simulink model "analiseLongitudinal_NL"  (R2016a)
settings: Solver=ode4  StartTime=0.0  StopTime=300  FixedStep=0.01  RelTol=1e-3
undefined symbols (not defined in the file): Ch, Ctheta, CVt, degtorad, Kh, Kq, Ktheta, KVt, Ue, Xe
libraries: simulink x13
settings Model: PauseTimes=50  Creator=Marcelo Henrique  LastModifiedBy=Marcelo
settings DataIOCC: LimitDataPoints=on  SaveFormat=Array
settings DebuggingCC: AlgebraicLoopMsg=none  UnderspecifiedInitializationDetection=Classic  MergeDetectMultiDrivingBlocksExec=none  StateNameClashWarn=warning
settings HardwareCC: ProdBitPerPointer=32  ProdLargestAtomicFloat=None  ProdIntDivRoundTo=Undefined  ProdEndianess=Unspecified  ProdWordSize=32  ProdHWDeviceType=32-bit Generic
settings ModelReferenceCC: PropagateSignalLabelsOutOfModel=off
settings RTWCC: CustomInclude=C:\Users\Marcelo\Desktop\cobem17\ctrl\matlab\mdl
settings ConfigComp: CovModelRefEnable=Off

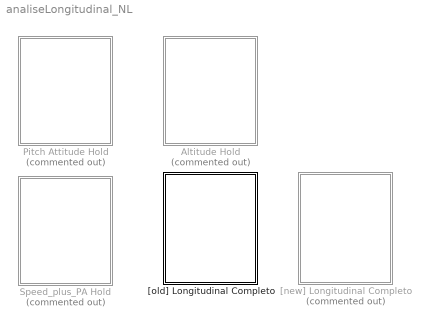
== system analiseLongitudinal_NL ==
  Altitude Hold : Subsystem  Commented=on
  Pitch Attitude Hold : Subsystem  Commented=on
  Speed_plus_PA Hold : Subsystem  Commented=on
  "[new] Longitudinal Completo" : Subsystem  Commented=on
  "[old] Longitudinal Completo" : Subsystem

== system analiseLongitudinal_NL/Altitude Hold ==
  Step1 : Step  Time=20  Before=-Xe(12)  After=-Xe(12)+5  SampleTime=0
  "[Aeronave]" : Subsystem
  "[Controle]" : Subsystem
  "[Navegação]" : Subsystem
  wires:
  "[Aeronave]"/1(Y) -> "[Navegação]"/1(Y)
  "[Navegação]"/1(Yn) -> "[Controle]"/2(Yn)
  Step1/1 -> "[Controle]"/1(Ref)
  "[Controle]"/1(du) -> "[Aeronave]"/1(du)

== system analiseLongitudinal_NL/Pitch Attitude Hold ==
  Step1 : Step  Time=20  Before=Xe(8)  After=degtorad(5)+(Xe(8))  SampleTime=0
  "[Aeronave]" : Subsystem
  "[Controle]" : Subsystem
  "[Navegação]" : Subsystem
  wires:
  "[Aeronave]"/1(Y) -> "[Navegação]"/1(Y)
  "[Controle]"/1(du) -> "[Aeronave]"/1(du)
  "[Navegação]"/1(Yn) -> "[Controle]"/2(Yn)
  Step1/1 -> "[Controle]"/1(Ref)

== system analiseLongitudinal_NL/Speed_plus_PA Hold ==
  Mux : Mux  Inputs=2
  VT_r : Step  Time=0  Before=norm(Xe(1:3))  After=norm(Xe(1:3))  SampleTime=0
  "[Aeronave]" : Subsystem
  "[Controle]" : Subsystem
  "[Navegação]" : Subsystem
  theta_r : Step  Time=20  Before=Xe(8)  After=degtorad(5)+(Xe(8))  SampleTime=0
  wires:
  "[Aeronave]"/1(Y) -> "[Navegação]"/1(Y)
  "[Controle]"/1(du) -> "[Aeronave]"/1(du)
  "[Navegação]"/1(Yn) -> "[Controle]"/2(Yn)
  VT_r/1 -> Mux/1
  theta_r/1 -> Mux/2
  Mux/1 -> "[Controle]"/1(Ref)

== system analiseLongitudinal_NL/[new] Longitudinal Completo ==
  Add : Sum  Inputs=+++
  Mux : Mux  Inputs=2
  Step : Step  Time=50  Before=-Xe(12)  After=-Xe(12)+40  SampleTime=0
  Step1 : Step  Time=150  After=-80  SampleTime=0
  Step2 : Step  Time=250  After=40  SampleTime=0
  Unit Delay : UnitDelay  SampleTime=-1
  VT_r : Step  Time=0  Before=norm(Xe(1:3))  After=norm(Xe(1:3))  SampleTime=0
  "[Aeronave]" : Subsystem
  "[Controle]" : Subsystem
  "[Navegação]" : Subsystem
  wires:
  VT_r/1 -> Mux/1
  Mux/1 -> "[Controle]"/1(U)
  "[Aeronave]"/1(Y) -> "[Navegação]"/1(Y)
  "[Controle]"/1(du) -> Unit Delay/1
  "[Navegação]"/1(Yn) -> "[Controle]"/2(Y)
  Add/1 -> Mux/2  "h_r"
  Step/1 -> Add/1
  Step1/1 -> Add/2
  Step2/1 -> Add/3
  Unit Delay/1 -> "[Aeronave]"/1(du)

== system analiseLongitudinal_NL/[old] Longitudinal Completo ==
  Add : Sum  Inputs=+++
  Mux : Mux  Inputs=2
  Step : Step  Time=50  Before=-Xe(12)  After=-Xe(12)+25  SampleTime=0
  Step1 : Step  Time=150  After=-50  SampleTime=0
  Step2 : Step  Time=250  After=25  SampleTime=0
  VT_r : Step  Time=0  Before=norm(Xe(1:3))  After=norm(Xe(1:3))  SampleTime=0
  "[Aeronave]" : Subsystem
  "[Controle]" : Subsystem
  "[Navegação]" : Subsystem
  wires:
  VT_r/1 -> Mux/1
  Mux/1 -> "[Controle]"/1(U)
  "[Aeronave]"/1(Y) -> "[Navegação]"/1(Y)
  "[Navegação]"/1(Yn) -> "[Controle]"/2(Y)
  Add/1 -> Mux/2  "h_r"
  Step/1 -> Add/1
  Step1/1 -> Add/2
  Step2/1 -> Add/3
  "[Controle]"/1(du) -> "[Aeronave]"/1(du)

== system analiseLongitudinal_NL/Altitude Hold/[Aeronave] ==
  du : Inport
  Entradas equilibrio : Constant  Value=Ue
  S-Function : S-Function  FunctionName=sfunction_piper  Parameters=par_gen,par_aero,par_prop, Xe  SFunctionDeploymentMode=off  EnableBusSupport=off
  Sum1 : Sum
  To Workspace1 : ToWorkspace  VariableName=NLU  SaveFormat=Timeseries  SampleTime=-1
  Y : Outport
  wires:
  S-Function/1 -> Y/1
  Entradas equilibrio/1 -> Sum1/2
  du/1 -> Sum1/1
  Sum1/1 -> To Workspace1/1, S-Function/1

== system analiseLongitudinal_NL/Altitude Hold/[Controle] ==
  Ref : Inport
  Yn : Inport  Port=2
  Controlador Elevator : Subsystem
  Gain8 : Gain  Gain=180/pi
  Mux : Mux
  To Workspace1 : ToWorkspace  VariableName=NLstep  SaveFormat=Timeseries  SampleTime=-1
  d_aileron : Constant  Value=0
  d_rudder : Constant  Value=0
  d_throttle : Constant  Value=0
  delta_e : Scope
  du : Outport
  wires:
  Yn/1 -> Controlador Elevator/2(Yn)
  Mux/1 -> du/1
  d_aileron/1 -> Mux/3
  d_rudder/1 -> Mux/4
  Gain8/1 -> delta_e/1
  Controlador Elevator/1(d_elevator) -> Gain8/1, Mux/2
  d_throttle/1 -> Mux/1
  Ref/1 -> To Workspace1/1, Controlador Elevator/1(h_r)

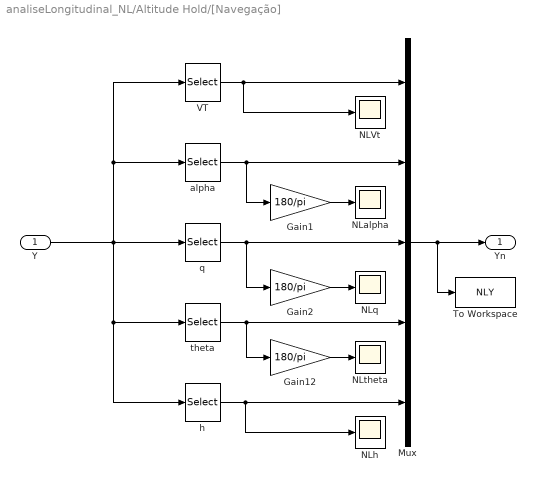
== system analiseLongitudinal_NL/Altitude Hold/[Navegação] ==
  Y : Inport
  Gain1 : Gain  Gain=180/pi
  Gain12 : Gain  Gain=180/pi
  Gain2 : Gain  Gain=180/pi
  Mux : Mux  Inputs=5
  NLVt : Scope
  NLalpha : Scope
  NLh : Scope
  NLq : Scope
  NLtheta : Scope
  To Workspace : ToWorkspace  VariableName=NLY  SaveFormat=Timeseries  SampleTime=-1
  VT : Selector  InputPortWidth=12  IndexOptions=Index vector (dialog)  Indices=[1]  OutputSizes=1
  alpha : Selector  InputPortWidth=12  IndexOptions=Index vector (dialog)  Indices=[2]  OutputSizes=1
  h : Selector  InputPortWidth=12  IndexOptions=Index vector (dialog)  Indices=[12]  OutputSizes=1
  q : Selector  InputPortWidth=12  IndexOptions=Index vector (dialog)  Indices=[5]  OutputSizes=1
  theta : Selector  InputPortWidth=12  IndexOptions=Index vector (dialog)  Indices=[8]  OutputSizes=1
  Yn : Outport
  wires:
  Y/1 -> h/1, theta/1, VT/1, alpha/1, q/1
  Gain12/1 -> NLtheta/1
  VT/1 -> NLVt/1, Mux/1
  theta/1 -> Gain12/1, Mux/4
  h/1 -> NLh/1, Mux/5
  Gain1/1 -> NLalpha/1
  alpha/1 -> Gain1/1, Mux/2
  Gain2/1 -> NLq/1
  q/1 -> Gain2/1, Mux/3
  Mux/1 -> To Workspace/1, Yn/1

== system analiseLongitudinal_NL/Pitch Attitude Hold/[Aeronave] ==
  du : Inport
  Entradas equilibrio : Constant  Value=Ue
  S-Function : S-Function  FunctionName=sfunction_piper  Parameters=par_gen,par_aero,par_prop, Xe  SFunctionDeploymentMode=off  EnableBusSupport=off
  Sum3 : Sum
  To Workspace1 : ToWorkspace  VariableName=NLU  SaveFormat=Timeseries  SampleTime=-1
  Y : Outport
  wires:
  Sum3/1 -> S-Function/1, To Workspace1/1
  du/1 -> Sum3/1
  S-Function/1 -> Y/1
  Entradas equilibrio/1 -> Sum3/2

== system analiseLongitudinal_NL/Pitch Attitude Hold/[Controle] ==
  Ref : Inport
  Yn : Inport  Port=2
  Controlador Elevator : Subsystem
  Gain8 : Gain  Gain=180/pi
  Mux : Mux
  To Workspace1 : ToWorkspace  VariableName=NLstep  SaveFormat=Timeseries  SampleTime=-1
  d_aileron : Constant  Value=0
  d_rudder : Constant  Value=0
  d_throttle : Constant  Value=0
  delta_e : Scope
  du : Outport
  wires:
  Yn/1 -> Controlador Elevator/2(Yn)
  Mux/1 -> du/1
  d_aileron/1 -> Mux/3
  d_rudder/1 -> Mux/4
  Gain8/1 -> delta_e/1
  Controlador Elevator/1(d_elevator) -> Gain8/1, Mux/2
  d_throttle/1 -> Mux/1
  Ref/1 -> To Workspace1/1, Controlador Elevator/1(theta_r)

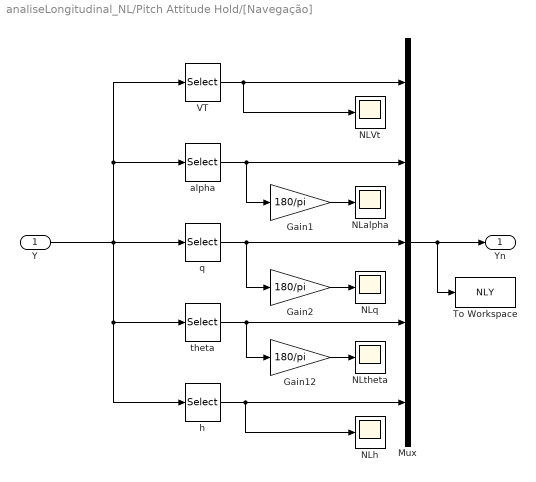
== system analiseLongitudinal_NL/Pitch Attitude Hold/[Navegação] ==
  Y : Inport
  Gain1 : Gain  Gain=180/pi
  Gain12 : Gain  Gain=180/pi
  Gain2 : Gain  Gain=180/pi
  Mux : Mux  Inputs=5
  NLVt : Scope
  NLalpha : Scope
  NLh : Scope
  NLq : Scope
  NLtheta : Scope
  To Workspace : ToWorkspace  VariableName=NLY  SaveFormat=Timeseries  SampleTime=-1
  VT : Selector  InputPortWidth=12  IndexOptions=Index vector (dialog)  Indices=[1]  OutputSizes=1
  alpha : Selector  InputPortWidth=12  IndexOptions=Index vector (dialog)  Indices=[2]  OutputSizes=1
  h : Selector  InputPortWidth=12  IndexOptions=Index vector (dialog)  Indices=[12]  OutputSizes=1
  q : Selector  InputPortWidth=12  IndexOptions=Index vector (dialog)  Indices=[5]  OutputSizes=1
  theta : Selector  InputPortWidth=12  IndexOptions=Index vector (dialog)  Indices=[8]  OutputSizes=1
  Yn : Outport
  wires:
  Y/1 -> h/1, theta/1, VT/1, alpha/1, q/1
  Gain12/1 -> NLtheta/1
  VT/1 -> NLVt/1, Mux/1
  theta/1 -> Gain12/1, Mux/4
  h/1 -> NLh/1, Mux/5
  Gain1/1 -> NLalpha/1
  alpha/1 -> Gain1/1, Mux/2
  Gain2/1 -> NLq/1
  q/1 -> Gain2/1, Mux/3
  Mux/1 -> To Workspace/1, Yn/1

== system analiseLongitudinal_NL/Speed_plus_PA Hold/[Aeronave] ==
  du : Inport
  Entradas equilibrio : Constant  Value=Ue
  S-Function : S-Function  FunctionName=sfunction_piper  Parameters=par_gen,par_aero,par_prop, Xe  SFunctionDeploymentMode=off  EnableBusSupport=off
  Sum1 : Sum
  To Workspace1 : ToWorkspace  VariableName=NLU  SaveFormat=Timeseries  SampleTime=-1
  Y : Outport
  wires:
  Sum1/1 -> To Workspace1/1, S-Function/1
  du/1 -> Sum1/1
  S-Function/1 -> Y/1
  Entradas equilibrio/1 -> Sum1/2

== system analiseLongitudinal_NL/Speed_plus_PA Hold/[Controle] ==
  Ref : Inport
  Yn : Inport  Port=2
  Controlador Elevator : Subsystem
  Controlador Throtle : Subsystem
  Mux : Mux
  To Workspace1 : ToWorkspace  VariableName=NLstep  SaveFormat=Timeseries  SampleTime=-1
  d_aileron : Constant  Value=0
  d_rudder : Constant  Value=0
  du : Outport
  wires:
  Mux/1 -> du/1
  d_aileron/1 -> Mux/3
  d_rudder/1 -> Mux/4
  Controlador Elevator/1(d_elevator) -> Mux/2
  Controlador Throtle/1(d_throtle) -> Mux/1
  Ref/1 -> To Workspace1/1, Controlador Elevator/1(theta_r), Controlador Throtle/1(Vt_r)
  Yn/1 -> Controlador Throtle/2(Yn), Controlador Elevator/2(Yn)

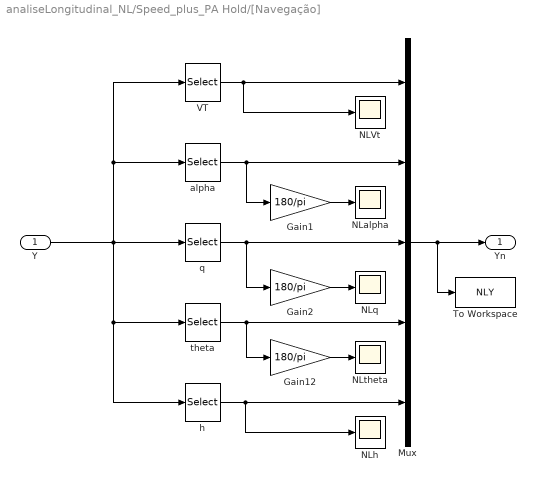
== system analiseLongitudinal_NL/Speed_plus_PA Hold/[Navegação] ==
  Y : Inport
  Gain1 : Gain  Gain=180/pi
  Gain12 : Gain  Gain=180/pi
  Gain2 : Gain  Gain=180/pi
  Mux : Mux  Inputs=5
  NLVt : Scope
  NLalpha : Scope
  NLh : Scope
  NLq : Scope
  NLtheta : Scope
  To Workspace : ToWorkspace  VariableName=NLY  SaveFormat=Timeseries  SampleTime=-1
  VT : Selector  InputPortWidth=12  IndexOptions=Index vector (dialog)  Indices=[1]  OutputSizes=1
  alpha : Selector  InputPortWidth=12  IndexOptions=Index vector (dialog)  Indices=[2]  OutputSizes=1
  h : Selector  InputPortWidth=12  IndexOptions=Index vector (dialog)  Indices=[12]  OutputSizes=1
  q : Selector  InputPortWidth=12  IndexOptions=Index vector (dialog)  Indices=[5]  OutputSizes=1
  theta : Selector  InputPortWidth=12  IndexOptions=Index vector (dialog)  Indices=[8]  OutputSizes=1
  Yn : Outport
  wires:
  Y/1 -> h/1, theta/1, VT/1, alpha/1, q/1
  Gain12/1 -> NLtheta/1
  VT/1 -> NLVt/1, Mux/1
  theta/1 -> Gain12/1, Mux/4
  h/1 -> NLh/1, Mux/5
  Gain1/1 -> NLalpha/1
  alpha/1 -> Gain1/1, Mux/2
  Gain2/1 -> NLq/1
  q/1 -> Gain2/1, Mux/3
  Mux/1 -> To Workspace/1, Yn/1

== system analiseLongitudinal_NL/[new] Longitudinal Completo/[Aeronave] ==
  du : Inport
  Entradas equilibrio : Constant  Value=Ue(1:4)
  S-Function : S-Function  FunctionName=sfunction_piper  Parameters=par_gen,par_aero,par_prop, Xe  SFunctionDeploymentMode=off  EnableBusSupport=off
  Sum3 : Sum
  To Workspace1 : ToWorkspace  VariableName=NLU_comp  SaveFormat=Timeseries  SampleTime=-1
  Y : Outport
  wires:
  du/1 -> Sum3/1
  Sum3/1 -> S-Function/1, To Workspace1/1
  S-Function/1 -> Y/1
  Entradas equilibrio/1 -> Sum3/2

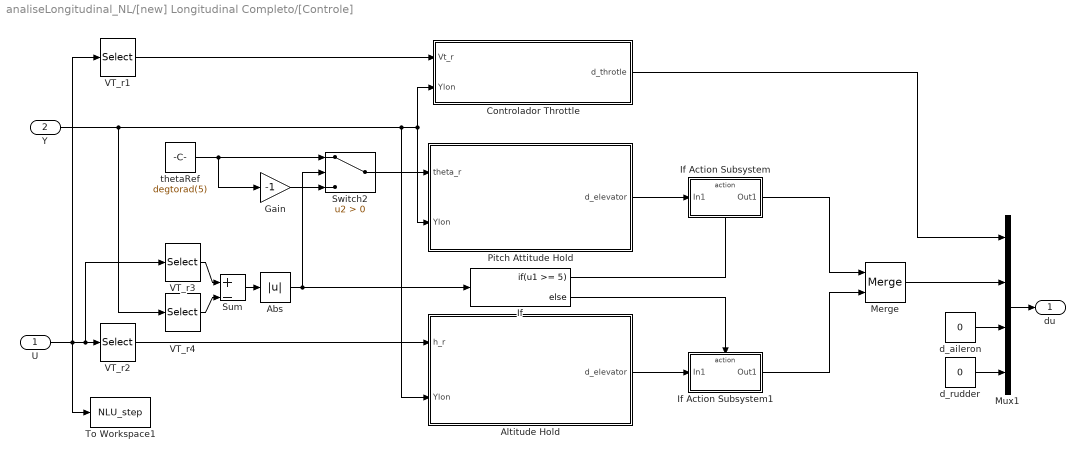
== system analiseLongitudinal_NL/[new] Longitudinal Completo/[Controle] ==
  U : Inport
  Y : Inport  Port=2
  Abs : Abs
  Altitude Hold : Subsystem
  Controlador Throttle : Subsystem
  Gain : Gain  Gain=-1
  If : If  IfExpression=u1 >= 5
  If Action Subsystem : Subsystem  TreatAsAtomicUnit=on
  If Action Subsystem1 : Subsystem  TreatAsAtomicUnit=on
  Merge : Merge
  Mux1 : Mux
  Pitch Attitude Hold : Subsystem
  Sum : Sum  Inputs=|+-
  Switch2 : Switch  Criteria=u2 > Threshold
  To Workspace1 : ToWorkspace  VariableName=NLU_step  SaveFormat=Timeseries  SampleTime=-1
  VT_r1 : Selector  InputPortWidth=2  IndexOptions=Index vector (dialog)  Indices=[1]  OutputSizes=1
  VT_r2 : Selector  InputPortWidth=2  IndexOptions=Index vector (dialog)  Indices=[2]  OutputSizes=1
  VT_r3 : Selector  InputPortWidth=2  IndexOptions=Index vector (dialog)  Indices=[2]  OutputSizes=1
  VT_r4 : Selector  InputPortWidth=5  IndexOptions=Index vector (dialog)  Indices=[5]  OutputSizes=1
  d_aileron : Constant  Value=0
  d_rudder : Constant  Value=0
  thetaRef : Constant  Value=degtorad(5)
  du : Outport
  wires:
  Mux1/1 -> du/1
  d_aileron/1 -> Mux1/3
  d_rudder/1 -> Mux1/4
  Gain/1 -> Switch2/3
  thetaRef/1 -> Gain/1, Switch2/1
  Switch2/1 -> Pitch Attitude Hold/1(theta_r)
  VT_r4/1 -> Sum/2
  Sum/1 -> Abs/1
  VT_r3/1 -> Sum/1
  Y/1 -> VT_r4/1, Altitude Hold/2(Ylon), Pitch Attitude Hold/2(Ylon), Controlador Throttle/2(Ylon)
  U/1 -> To Workspace1/1, VT_r3/1, VT_r2/1, VT_r1/1
  VT_r2/1 -> Altitude Hold/1(h_r)
  VT_r1/1 -> Controlador Throttle/1(Vt_r)
  Abs/1 -> If/1, Switch2/2
  Pitch Attitude Hold/1(d_elevator) -> If Action Subsystem/1(In1)
  If Action Subsystem/1(Out1) -> Merge/1
  If/1 -> If Action Subsystem/Action
  If Action Subsystem1/1(Out1) -> Merge/2
  Altitude Hold/1(d_elevator) -> If Action Subsystem1/1(In1)
  If/2 -> If Action Subsystem1/Action
  Controlador Throttle/1(d_throtle) -> Mux1/1
  Merge/1 -> Mux1/2

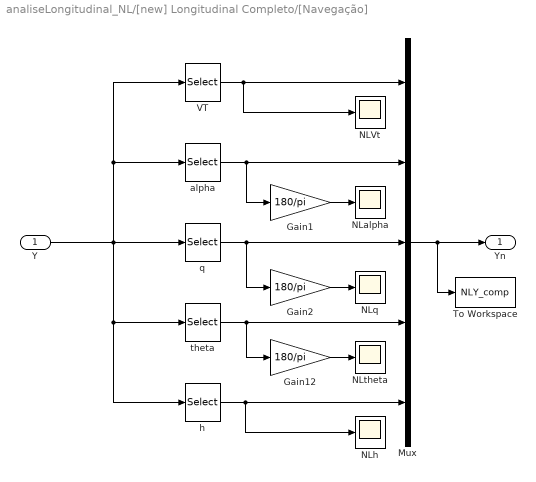
== system analiseLongitudinal_NL/[new] Longitudinal Completo/[Navegação] ==
  Y : Inport
  Gain1 : Gain  Gain=180/pi
  Gain12 : Gain  Gain=180/pi
  Gain2 : Gain  Gain=180/pi
  Mux : Mux  Inputs=5
  NLVt : Scope
  NLalpha : Scope
  NLh : Scope
  NLq : Scope
  NLtheta : Scope
  To Workspace : ToWorkspace  VariableName=NLY_comp  SaveFormat=Timeseries  SampleTime=-1
  VT : Selector  InputPortWidth=12  IndexOptions=Index vector (dialog)  Indices=[1]  OutputSizes=1
  alpha : Selector  InputPortWidth=12  IndexOptions=Index vector (dialog)  Indices=[2]  OutputSizes=1
  h : Selector  InputPortWidth=12  IndexOptions=Index vector (dialog)  Indices=[12]  OutputSizes=1
  q : Selector  InputPortWidth=12  IndexOptions=Index vector (dialog)  Indices=[5]  OutputSizes=1
  theta : Selector  InputPortWidth=12  IndexOptions=Index vector (dialog)  Indices=[8]  OutputSizes=1
  Yn : Outport
  wires:
  Y/1 -> h/1, theta/1, VT/1, alpha/1, q/1
  Gain12/1 -> NLtheta/1
  VT/1 -> NLVt/1, Mux/1
  theta/1 -> Gain12/1, Mux/4
  h/1 -> NLh/1, Mux/5
  Gain1/1 -> NLalpha/1
  alpha/1 -> Gain1/1, Mux/2
  Gain2/1 -> NLq/1
  q/1 -> Gain2/1, Mux/3
  Mux/1 -> To Workspace/1, Yn/1

== system analiseLongitudinal_NL/[old] Longitudinal Completo/[Aeronave] ==
  du : Inport
  Entradas equilibrio : Constant  Value=Ue(1:4)
  S-Function : S-Function  FunctionName=sfunction_piper  Parameters=par_gen,par_aero,par_prop, Xe  SFunctionDeploymentMode=off  EnableBusSupport=off
  Sum3 : Sum
  To Workspace1 : ToWorkspace  VariableName=NLU  SaveFormat=Timeseries  SampleTime=-1
  Y : Outport
  wires:
  du/1 -> Sum3/1
  Sum3/1 -> S-Function/1, To Workspace1/1
  Entradas equilibrio/1 -> Sum3/2
  S-Function/1 -> Y/1

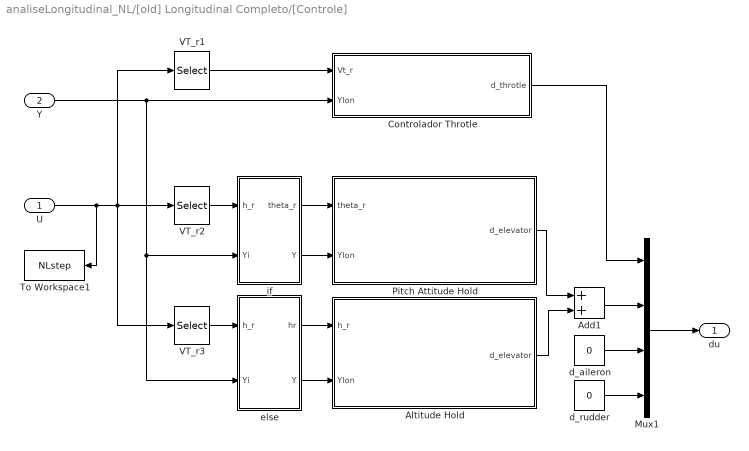
== system analiseLongitudinal_NL/[old] Longitudinal Completo/[Controle] ==
  U : Inport
  Y : Inport  Port=2
  Add1 : Sum
  Altitude Hold : Subsystem
  Controlador Throtle : Subsystem
  Mux1 : Mux
  Pitch Attitude Hold : Subsystem
  To Workspace1 : ToWorkspace  VariableName=NLstep  SaveFormat=Timeseries  SampleTime=-1
  VT_r1 : Selector  InputPortWidth=2  IndexOptions=Index vector (dialog)  Indices=[1]  OutputSizes=1
  VT_r2 : Selector  InputPortWidth=2  IndexOptions=Index vector (dialog)  Indices=[2]  OutputSizes=1
  VT_r3 : Selector  InputPortWidth=2  IndexOptions=Index vector (dialog)  Indices=[2]  OutputSizes=1
  d_aileron : Constant  Value=0
  d_rudder : Constant  Value=0
  else : Subsystem
  if : Subsystem
  du : Outport
  wires:
  Pitch Attitude Hold/1(d_elevator) -> Add1/1
  Controlador Throtle/1(d_throtle) -> Mux1/1
  Altitude Hold/1(d_elevator) -> Add1/2
  Mux1/1 -> du/1
  if/2(Y) -> Pitch Attitude Hold/2(Ylon)
  Add1/1 -> Mux1/2
  if/1(theta_r) -> Pitch Attitude Hold/1(theta_r)
  else/2(Y) -> Altitude Hold/2(Ylon)
  else/1(hr) -> Altitude Hold/1(h_r)
  VT_r3/1 -> else/1(h_r)
  VT_r2/1 -> if/1(h_r)
  VT_r1/1 -> Controlador Throtle/1(Vt_r)
  Y/1 -> if/2(Yi), else/2(Yi), Controlador Throtle/2(Ylon)
  d_aileron/1 -> Mux1/3
  d_rudder/1 -> Mux1/4
  U/1 -> To Workspace1/1, VT_r1/1, VT_r3/1, VT_r2/1

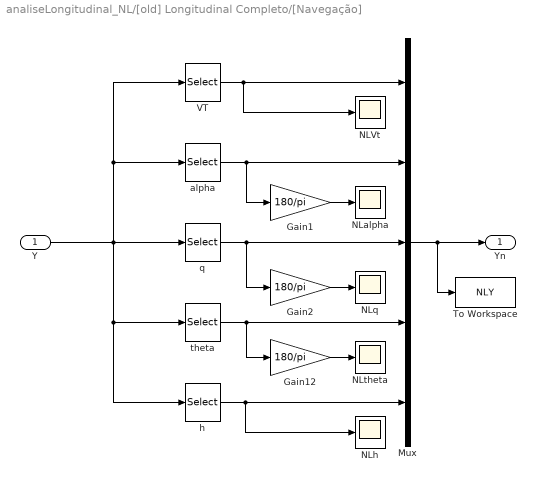
== system analiseLongitudinal_NL/[old] Longitudinal Completo/[Navegação] ==
  Y : Inport
  Gain1 : Gain  Gain=180/pi
  Gain12 : Gain  Gain=180/pi
  Gain2 : Gain  Gain=180/pi
  Mux : Mux  Inputs=5
  NLVt : Scope
  NLalpha : Scope
  NLh : Scope
  NLq : Scope
  NLtheta : Scope
  To Workspace : ToWorkspace  VariableName=NLY  SaveFormat=Timeseries  SampleTime=-1
  VT : Selector  InputPortWidth=12  IndexOptions=Index vector (dialog)  Indices=[1]  OutputSizes=1
  alpha : Selector  InputPortWidth=12  IndexOptions=Index vector (dialog)  Indices=[2]  OutputSizes=1
  h : Selector  InputPortWidth=12  IndexOptions=Index vector (dialog)  Indices=[12]  OutputSizes=1
  q : Selector  InputPortWidth=12  IndexOptions=Index vector (dialog)  Indices=[5]  OutputSizes=1
  theta : Selector  InputPortWidth=12  IndexOptions=Index vector (dialog)  Indices=[8]  OutputSizes=1
  Yn : Outport
  wires:
  Y/1 -> h/1, theta/1, VT/1, alpha/1, q/1
  Gain12/1 -> NLtheta/1
  VT/1 -> NLVt/1, Mux/1
  theta/1 -> Gain12/1, Mux/4
  h/1 -> NLh/1, Mux/5
  Gain1/1 -> NLalpha/1
  alpha/1 -> Gain1/1, Mux/2
  Gain2/1 -> NLq/1
  q/1 -> Gain2/1, Mux/3
  Mux/1 -> To Workspace/1, Yn/1

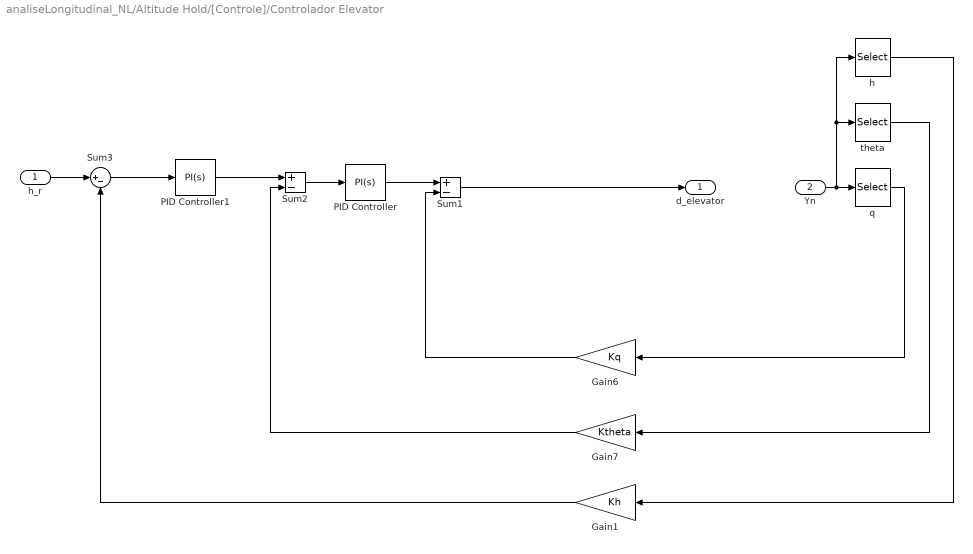
== system analiseLongitudinal_NL/Altitude Hold/[Controle]/Controlador Elevator ==
  h_r : Inport
  Yn : Inport  Port=2
  Gain1 : Gain  Gain=Kh
  Gain6 : Gain  Gain=Kq
  Gain7 : Gain  Gain=Ktheta
  PID Controller : simulink/Continuous/PID Controller  Controller=PI  TimeDomain=Continuous-time  SampleTime=-1  IntegratorMethod=Forward Euler  FilterMethod=Forward Euler  Form=Parallel  UseFilter=on  ControllerParametersSource=internal  P=Ctheta.Kp  I=Ctheta.Ki  D=0  N=100  InitialConditionSource=internal  InitialConditionForIntegrator=0  InitialConditionForFilter=0  ExternalReset=none  LimitOutput=off  UpperSaturationLimit=inf  LowerSaturationLimit=-inf  LinearizeAsGain=on  AntiWindupMode=none  Kb=1  TrackingMode=off  Kt=1  PParamMin=[]  PParamMax=[]  IParamMin=[]  IParamMax=[]  DParamMin=[]  DParamMax=[]  NParamMin=[]  NParamMax=[]  KbParamMin=[]  KbParamMax=[]  KtParamMin=[]  KtParamMax=[]  POutMin=[]  POutMax=[]  IOutMin=[]  IOutMax=[]  DOutMin=[]  DOutMax=[]  NOutMin=[]  NOutMax=[]  KbOutMin=[]  KbOutMax=[]  KtOutMin=[]  KtOutMax=[]  IntegratorOutMin=[]  IntegratorOutMax=[]  FilterOutMin=[]  FilterOutMax=[]  SumOutMin=[]  SumOutMax=[]  SumI1OutMin=[]  SumI1OutMax=[]  SumI2OutMin=[]  SumI2OutMax=[]  SumI3OutMin=[]  SumI3OutMax=[]  SumDOutMin=[]  SumDOutMax=[]  SaturationOutMin=[]  SaturationOutMax=[]  IntegratorContinuousStateAttributes=''  IntegratorStateMustResolveToSignalObject=off  IntegratorRTWStateStorageClass=Auto  FilterContinuousStateAttributes=''  FilterStateMustResolveToSignalObject=off  FilterRTWStateStorageClass=Auto  DifferentiatorICPrevScaledInput=0  DifferentiatorOutMin=[]  DifferentiatorOutMax=[]
  PID Controller1 : simulink/Continuous/PID Controller  Controller=PI  TimeDomain=Continuous-time  SampleTime=-1  IntegratorMethod=Forward Euler  FilterMethod=Forward Euler  Form=Parallel  UseFilter=on  ControllerParametersSource=internal  P=Ch.Kp  I=Ch.Ki  D=0  N=100  InitialConditionSource=internal  InitialConditionForIntegrator=0  InitialConditionForFilter=0  ExternalReset=none  LimitOutput=off  UpperSaturationLimit=inf  LowerSaturationLimit=-inf  LinearizeAsGain=on  AntiWindupMode=none  Kb=1  TrackingMode=off  Kt=1  PParamMin=[]  PParamMax=[]  IParamMin=[]  IParamMax=[]  DParamMin=[]  DParamMax=[]  NParamMin=[]  NParamMax=[]  KbParamMin=[]  KbParamMax=[]  KtParamMin=[]  KtParamMax=[]  POutMin=[]  POutMax=[]  IOutMin=[]  IOutMax=[]  DOutMin=[]  DOutMax=[]  NOutMin=[]  NOutMax=[]  KbOutMin=[]  KbOutMax=[]  KtOutMin=[]  KtOutMax=[]  IntegratorOutMin=[]  IntegratorOutMax=[]  FilterOutMin=[]  FilterOutMax=[]  SumOutMin=[]  SumOutMax=[]  SumI1OutMin=[]  SumI1OutMax=[]  SumI2OutMin=[]  SumI2OutMax=[]  SumI3OutMin=[]  SumI3OutMax=[]  SumDOutMin=[]  SumDOutMax=[]  SaturationOutMin=[]  SaturationOutMax=[]  IntegratorContinuousStateAttributes=''  IntegratorStateMustResolveToSignalObject=off  IntegratorRTWStateStorageClass=Auto  FilterContinuousStateAttributes=''  FilterStateMustResolveToSignalObject=off  FilterRTWStateStorageClass=Auto  DifferentiatorICPrevScaledInput=0  DifferentiatorOutMin=[]  DifferentiatorOutMax=[]
  Sum1 : Sum  Inputs=+-
  Sum2 : Sum  Inputs=+-
  Sum3 : Sum  Inputs=|+-
  h : Selector  InputPortWidth=5  IndexOptions=Index vector (dialog)  Indices=[5]  OutputSizes=1
  q : Selector  InputPortWidth=5  IndexOptions=Index vector (dialog)  Indices=[3]  OutputSizes=1
  theta : Selector  InputPortWidth=5  IndexOptions=Index vector (dialog)  Indices=[4]  OutputSizes=1
  d_elevator : Outport
  wires:
  theta/1 -> Gain7/1
  q/1 -> Gain6/1
  Gain6/1 -> Sum1/2
  Gain7/1 -> Sum2/2
  PID Controller/1 -> Sum1/1
  Sum2/1 -> PID Controller/1
  Yn/1 -> h/1, theta/1, q/1
  Gain1/1 -> Sum3/2
  h_r/1 -> Sum3/1
  Sum3/1 -> PID Controller1/1
  PID Controller1/1 -> Sum2/1
  h/1 -> Gain1/1
  Sum1/1 -> d_elevator/1

== system analiseLongitudinal_NL/Pitch Attitude Hold/[Controle]/Controlador Elevator ==
  theta_r : Inport
  Yn : Inport  Port=2
  Gain6 : Gain  Gain=Kq
  Gain7 : Gain  Gain=Ktheta
  PID Controller : simulink/Continuous/PID Controller  Controller=PI  TimeDomain=Continuous-time  SampleTime=-1  IntegratorMethod=Forward Euler  FilterMethod=Forward Euler  Form=Parallel  UseFilter=on  ControllerParametersSource=internal  P=Ctheta.Kp  I=Ctheta.Ki  D=0  N=100  InitialConditionSource=internal  InitialConditionForIntegrator=0  InitialConditionForFilter=0  ExternalReset=none  LimitOutput=off  UpperSaturationLimit=inf  LowerSaturationLimit=-inf  LinearizeAsGain=on  AntiWindupMode=none  Kb=1  TrackingMode=off  Kt=1  PParamMin=[]  PParamMax=[]  IParamMin=[]  IParamMax=[]  DParamMin=[]  DParamMax=[]  NParamMin=[]  NParamMax=[]  KbParamMin=[]  KbParamMax=[]  KtParamMin=[]  KtParamMax=[]  POutMin=[]  POutMax=[]  IOutMin=[]  IOutMax=[]  DOutMin=[]  DOutMax=[]  NOutMin=[]  NOutMax=[]  KbOutMin=[]  KbOutMax=[]  KtOutMin=[]  KtOutMax=[]  IntegratorOutMin=[]  IntegratorOutMax=[]  FilterOutMin=[]  FilterOutMax=[]  SumOutMin=[]  SumOutMax=[]  SumI1OutMin=[]  SumI1OutMax=[]  SumI2OutMin=[]  SumI2OutMax=[]  SumI3OutMin=[]  SumI3OutMax=[]  SumDOutMin=[]  SumDOutMax=[]  SaturationOutMin=[]  SaturationOutMax=[]  IntegratorContinuousStateAttributes=''  IntegratorStateMustResolveToSignalObject=off  IntegratorRTWStateStorageClass=Auto  FilterContinuousStateAttributes=''  FilterStateMustResolveToSignalObject=off  FilterRTWStateStorageClass=Auto  DifferentiatorICPrevScaledInput=0  DifferentiatorOutMin=[]  DifferentiatorOutMax=[]
  Sum1 : Sum  Inputs=+-
  Sum2 : Sum  Inputs=+-
  q : Selector  InputPortWidth=5  IndexOptions=Index vector (dialog)  Indices=[3]  OutputSizes=1
  theta : Selector  InputPortWidth=5  IndexOptions=Index vector (dialog)  Indices=[4]  OutputSizes=1
  d_elevator : Outport
  wires:
  theta/1 -> Gain7/1
  q/1 -> Gain6/1
  Gain6/1 -> Sum1/2
  Gain7/1 -> Sum2/2
  PID Controller/1 -> Sum1/1
  Sum2/1 -> PID Controller/1
  theta_r/1 -> Sum2/1
  Yn/1 -> theta/1, q/1
  Sum1/1 -> d_elevator/1

== system analiseLongitudinal_NL/Speed_plus_PA Hold/[Controle]/Controlador Elevator ==
  theta_r : Inport
  Yn : Inport  Port=2
  Gain6 : Gain  Gain=Kq
  Gain7 : Gain  Gain=Ktheta
  PID Controller : simulink/Continuous/PID Controller  Controller=PI  TimeDomain=Continuous-time  SampleTime=-1  IntegratorMethod=Forward Euler  FilterMethod=Forward Euler  Form=Parallel  UseFilter=on  ControllerParametersSource=internal  P=Ctheta.Kp  I=Ctheta.Ki  D=0  N=100  InitialConditionSource=internal  InitialConditionForIntegrator=0  InitialConditionForFilter=0  ExternalReset=none  LimitOutput=off  UpperSaturationLimit=inf  LowerSaturationLimit=-inf  LinearizeAsGain=on  AntiWindupMode=none  Kb=1  TrackingMode=off  Kt=1  PParamMin=[]  PParamMax=[]  IParamMin=[]  IParamMax=[]  DParamMin=[]  DParamMax=[]  NParamMin=[]  NParamMax=[]  KbParamMin=[]  KbParamMax=[]  KtParamMin=[]  KtParamMax=[]  POutMin=[]  POutMax=[]  IOutMin=[]  IOutMax=[]  DOutMin=[]  DOutMax=[]  NOutMin=[]  NOutMax=[]  KbOutMin=[]  KbOutMax=[]  KtOutMin=[]  KtOutMax=[]  IntegratorOutMin=[]  IntegratorOutMax=[]  FilterOutMin=[]  FilterOutMax=[]  SumOutMin=[]  SumOutMax=[]  SumI1OutMin=[]  SumI1OutMax=[]  SumI2OutMin=[]  SumI2OutMax=[]  SumI3OutMin=[]  SumI3OutMax=[]  SumDOutMin=[]  SumDOutMax=[]  SaturationOutMin=[]  SaturationOutMax=[]  IntegratorContinuousStateAttributes=''  IntegratorStateMustResolveToSignalObject=off  IntegratorRTWStateStorageClass=Auto  FilterContinuousStateAttributes=''  FilterStateMustResolveToSignalObject=off  FilterRTWStateStorageClass=Auto  DifferentiatorICPrevScaledInput=0  DifferentiatorOutMin=[]  DifferentiatorOutMax=[]
  Saturation : Saturate  UpperLimit=15*pi/180  LowerLimit=-15*pi/180
  Sum1 : Sum  Inputs=+-
  Sum2 : Sum  Inputs=+-
  h_r1 : Selector  InputPortWidth=2  IndexOptions=Index vector (dialog)  Indices=[2]  OutputSizes=1
  q : Selector  InputPortWidth=5  IndexOptions=Index vector (dialog)  Indices=[3]  OutputSizes=1
  theta : Selector  InputPortWidth=5  IndexOptions=Index vector (dialog)  Indices=[4]  OutputSizes=1
  d_elevator : Outport
  wires:
  theta/1 -> Gain7/1
  q/1 -> Gain6/1
  Gain6/1 -> Sum1/2
  Gain7/1 -> Sum2/2
  PID Controller/1 -> Sum1/1
  Sum2/1 -> PID Controller/1
  Yn/1 -> theta/1, q/1
  Saturation/1 -> d_elevator/1
  Sum1/1 -> Saturation/1
  theta_r/1 -> h_r1/1
  h_r1/1 -> Sum2/1

== system analiseLongitudinal_NL/Speed_plus_PA Hold/[Controle]/Controlador Throtle ==
  Vt_r : Inport
  Yn : Inport  Port=2
  Gain7 : Gain  Gain=KVt
  PID Controller1 : simulink/Continuous/PID Controller  Controller=PI  TimeDomain=Continuous-time  SampleTime=-1  IntegratorMethod=Forward Euler  FilterMethod=Forward Euler  Form=Parallel  UseFilter=on  ControllerParametersSource=internal  P=CVt.Kp  I=CVt.Ki  D=0  N=100  InitialConditionSource=internal  InitialConditionForIntegrator=0  InitialConditionForFilter=0  ExternalReset=none  LimitOutput=off  UpperSaturationLimit=inf  LowerSaturationLimit=-inf  LinearizeAsGain=on  AntiWindupMode=none  Kb=1  TrackingMode=off  Kt=1  PParamMin=[]  PParamMax=[]  IParamMin=[]  IParamMax=[]  DParamMin=[]  DParamMax=[]  NParamMin=[]  NParamMax=[]  KbParamMin=[]  KbParamMax=[]  KtParamMin=[]  KtParamMax=[]  POutMin=[]  POutMax=[]  IOutMin=[]  IOutMax=[]  DOutMin=[]  DOutMax=[]  NOutMin=[]  NOutMax=[]  KbOutMin=[]  KbOutMax=[]  KtOutMin=[]  KtOutMax=[]  IntegratorOutMin=[]  IntegratorOutMax=[]  FilterOutMin=[]  FilterOutMax=[]  SumOutMin=[]  SumOutMax=[]  SumI1OutMin=[]  SumI1OutMax=[]  SumI2OutMin=[]  SumI2OutMax=[]  SumI3OutMin=[]  SumI3OutMax=[]  SumDOutMin=[]  SumDOutMax=[]  SaturationOutMin=[]  SaturationOutMax=[]  IntegratorContinuousStateAttributes=''  IntegratorStateMustResolveToSignalObject=off  IntegratorRTWStateStorageClass=Auto  FilterContinuousStateAttributes=''  FilterStateMustResolveToSignalObject=off  FilterRTWStateStorageClass=Auto  DifferentiatorICPrevScaledInput=0  DifferentiatorOutMin=[]  DifferentiatorOutMax=[]
  Sum : Sum  Inputs=+-
  VT : Selector  InputPortWidth=5  IndexOptions=Index vector (dialog)  Indices=1  OutputSizes=1
  VT_r : Selector  InputPortWidth=2  IndexOptions=Index vector (dialog)  Indices=[1]  OutputSizes=1
  d_throtle : Outport
  wires:
  Vt_r/1 -> VT_r/1
  Sum/1 -> PID Controller1/1
  VT_r/1 -> Sum/1
  Yn/1 -> VT/1
  VT/1 -> Gain7/1
  Gain7/1 -> Sum/2
  PID Controller1/1 -> d_throtle/1

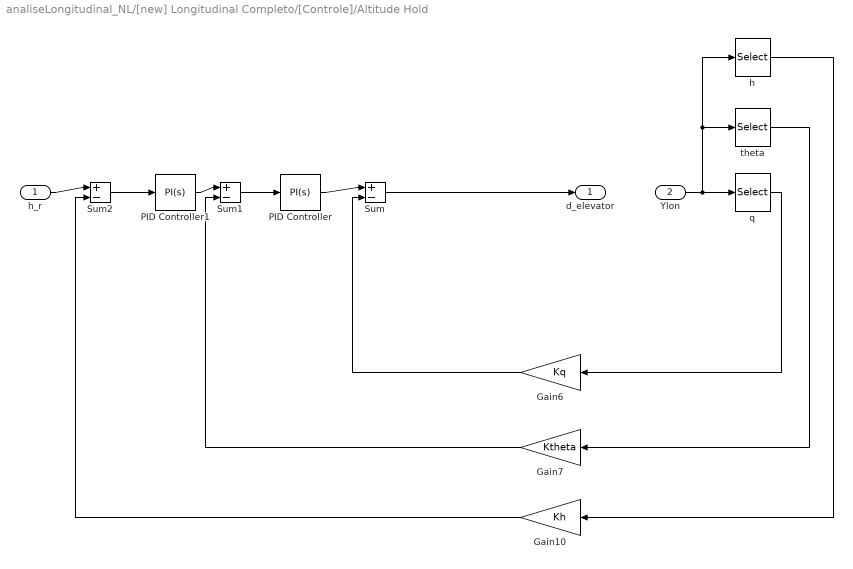
== system analiseLongitudinal_NL/[new] Longitudinal Completo/[Controle]/Altitude Hold ==
  h_r : Inport
  Ylon : Inport  Port=2
  Gain10 : Gain  Gain=Kh
  Gain6 : Gain  Gain=Kq
  Gain7 : Gain  Gain=Ktheta
  PID Controller : simulink/Continuous/PID Controller  Controller=PI  TimeDomain=Continuous-time  SampleTime=-1  IntegratorMethod=Forward Euler  FilterMethod=Forward Euler  Form=Parallel  UseFilter=on  ControllerParametersSource=internal  P=Ctheta.Kp  I=Ctheta.Ki  D=0  N=100  InitialConditionSource=internal  InitialConditionForIntegrator=0  InitialConditionForFilter=0  ExternalReset=none  LimitOutput=off  UpperSaturationLimit=inf  LowerSaturationLimit=-inf  LinearizeAsGain=on  AntiWindupMode=none  Kb=1  TrackingMode=off  Kt=1  PParamMin=[]  PParamMax=[]  IParamMin=[]  IParamMax=[]  DParamMin=[]  DParamMax=[]  NParamMin=[]  NParamMax=[]  KbParamMin=[]  KbParamMax=[]  KtParamMin=[]  KtParamMax=[]  POutMin=[]  POutMax=[]  IOutMin=[]  IOutMax=[]  DOutMin=[]  DOutMax=[]  NOutMin=[]  NOutMax=[]  KbOutMin=[]  KbOutMax=[]  KtOutMin=[]  KtOutMax=[]  IntegratorOutMin=[]  IntegratorOutMax=[]  FilterOutMin=[]  FilterOutMax=[]  SumOutMin=[]  SumOutMax=[]  SumI1OutMin=[]  SumI1OutMax=[]  SumI2OutMin=[]  SumI2OutMax=[]  SumI3OutMin=[]  SumI3OutMax=[]  SumDOutMin=[]  SumDOutMax=[]  SaturationOutMin=[]  SaturationOutMax=[]  IntegratorContinuousStateAttributes=''  IntegratorStateMustResolveToSignalObject=off  IntegratorRTWStateStorageClass=Auto  FilterContinuousStateAttributes=''  FilterStateMustResolveToSignalObject=off  FilterRTWStateStorageClass=Auto  DifferentiatorICPrevScaledInput=0  DifferentiatorOutMin=[]  DifferentiatorOutMax=[]
  PID Controller1 : simulink/Continuous/PID Controller  Controller=PI  TimeDomain=Continuous-time  SampleTime=-1  IntegratorMethod=Forward Euler  FilterMethod=Forward Euler  Form=Parallel  UseFilter=on  ControllerParametersSource=internal  P=Ch.Kp  I=Ch.Ki  D=0  N=100  InitialConditionSource=internal  InitialConditionForIntegrator=0  InitialConditionForFilter=0  ExternalReset=none  LimitOutput=off  UpperSaturationLimit=inf  LowerSaturationLimit=-inf  LinearizeAsGain=on  AntiWindupMode=none  Kb=1  TrackingMode=off  Kt=1  PParamMin=[]  PParamMax=[]  IParamMin=[]  IParamMax=[]  DParamMin=[]  DParamMax=[]  NParamMin=[]  NParamMax=[]  KbParamMin=[]  KbParamMax=[]  KtParamMin=[]  KtParamMax=[]  POutMin=[]  POutMax=[]  IOutMin=[]  IOutMax=[]  DOutMin=[]  DOutMax=[]  NOutMin=[]  NOutMax=[]  KbOutMin=[]  KbOutMax=[]  KtOutMin=[]  KtOutMax=[]  IntegratorOutMin=[]  IntegratorOutMax=[]  FilterOutMin=[]  FilterOutMax=[]  SumOutMin=[]  SumOutMax=[]  SumI1OutMin=[]  SumI1OutMax=[]  SumI2OutMin=[]  SumI2OutMax=[]  SumI3OutMin=[]  SumI3OutMax=[]  SumDOutMin=[]  SumDOutMax=[]  SaturationOutMin=[]  SaturationOutMax=[]  IntegratorContinuousStateAttributes=''  IntegratorStateMustResolveToSignalObject=off  IntegratorRTWStateStorageClass=Auto  FilterContinuousStateAttributes=''  FilterStateMustResolveToSignalObject=off  FilterRTWStateStorageClass=Auto  DifferentiatorICPrevScaledInput=0  DifferentiatorOutMin=[]  DifferentiatorOutMax=[]
  Sum : Sum  Inputs=|+-
  Sum1 : Sum  Inputs=|+-
  Sum2 : Sum  Inputs=|+-
  h : Selector  InputPortWidth=5  IndexOptions=Index vector (dialog)  Indices=[5]  OutputSizes=1
  q : Selector  InputPortWidth=5  IndexOptions=Index vector (dialog)  Indices=[3]  OutputSizes=1
  theta : Selector  InputPortWidth=5  IndexOptions=Index vector (dialog)  Indices=[4]  OutputSizes=1
  d_elevator : Outport
  wires:
  Gain6/1 -> Sum/2
  Gain7/1 -> Sum1/2
  PID Controller/1 -> Sum/1
  Sum1/1 -> PID Controller/1
  PID Controller1/1 -> Sum1/1
  Gain10/1 -> Sum2/2
  Sum2/1 -> PID Controller1/1
  theta/1 -> Gain7/1
  q/1 -> Gain6/1
  Ylon/1 -> theta/1, h/1, q/1
  h/1 -> Gain10/1
  Sum/1 -> d_elevator/1
  h_r/1 -> Sum2/1

== system analiseLongitudinal_NL/[new] Longitudinal Completo/[Controle]/Controlador Throttle ==
  Vt_r : Inport
  Ylon : Inport  Port=2
  Gain7 : Gain  Gain=KVt
  PID Controller1 : simulink/Continuous/PID Controller  Controller=PI  TimeDomain=Continuous-time  SampleTime=-1  IntegratorMethod=Forward Euler  FilterMethod=Forward Euler  Form=Parallel  UseFilter=on  ControllerParametersSource=internal  P=CVt.Kp  I=CVt.Ki  D=0  N=100  InitialConditionSource=internal  InitialConditionForIntegrator=0  InitialConditionForFilter=0  ExternalReset=none  LimitOutput=off  UpperSaturationLimit=inf  LowerSaturationLimit=-inf  LinearizeAsGain=on  AntiWindupMode=none  Kb=1  TrackingMode=off  Kt=1  PParamMin=[]  PParamMax=[]  IParamMin=[]  IParamMax=[]  DParamMin=[]  DParamMax=[]  NParamMin=[]  NParamMax=[]  KbParamMin=[]  KbParamMax=[]  KtParamMin=[]  KtParamMax=[]  POutMin=[]  POutMax=[]  IOutMin=[]  IOutMax=[]  DOutMin=[]  DOutMax=[]  NOutMin=[]  NOutMax=[]  KbOutMin=[]  KbOutMax=[]  KtOutMin=[]  KtOutMax=[]  IntegratorOutMin=[]  IntegratorOutMax=[]  FilterOutMin=[]  FilterOutMax=[]  SumOutMin=[]  SumOutMax=[]  SumI1OutMin=[]  SumI1OutMax=[]  SumI2OutMin=[]  SumI2OutMax=[]  SumI3OutMin=[]  SumI3OutMax=[]  SumDOutMin=[]  SumDOutMax=[]  SaturationOutMin=[]  SaturationOutMax=[]  IntegratorContinuousStateAttributes=''  IntegratorStateMustResolveToSignalObject=off  IntegratorRTWStateStorageClass=Auto  FilterContinuousStateAttributes=''  FilterStateMustResolveToSignalObject=off  FilterRTWStateStorageClass=Auto  DifferentiatorICPrevScaledInput=0  DifferentiatorOutMin=[]  DifferentiatorOutMax=[]
  Sum : Sum  Inputs=+-
  VT : Selector  InputPortWidth=5  IndexOptions=Index vector (dialog)  Indices=1  OutputSizes=1
  d_throtle : Outport
  wires:
  Sum/1 -> PID Controller1/1
  Vt_r/1 -> Sum/1
  Ylon/1 -> VT/1
  VT/1 -> Gain7/1
  Gain7/1 -> Sum/2
  PID Controller1/1 -> d_throtle/1

== system analiseLongitudinal_NL/[new] Longitudinal Completo/[Controle]/If Action Subsystem ==
  In1 : Inport
  Action Port : ActionPort  ActionType=then
  Out1 : Outport
  wires:
  In1/1 -> Out1/1

== system analiseLongitudinal_NL/[new] Longitudinal Completo/[Controle]/If Action Subsystem1 ==
  In1 : Inport
  Action Port : ActionPort  ActionType=else
  Out1 : Outport
  wires:
  In1/1 -> Out1/1

== system analiseLongitudinal_NL/[new] Longitudinal Completo/[Controle]/Pitch Attitude Hold ==
  theta_r : Inport
  Ylon : Inport  Port=2
  Gain6 : Gain  Gain=Kq
  Gain7 : Gain  Gain=Ktheta
  PID Controller : simulink/Continuous/PID Controller  Controller=PI  TimeDomain=Continuous-time  SampleTime=-1  IntegratorMethod=Forward Euler  FilterMethod=Forward Euler  Form=Parallel  UseFilter=on  ControllerParametersSource=internal  P=Ctheta.Kp  I=Ctheta.Ki  D=0  N=100  InitialConditionSource=internal  InitialConditionForIntegrator=0  InitialConditionForFilter=0  ExternalReset=none  LimitOutput=off  UpperSaturationLimit=inf  LowerSaturationLimit=-inf  LinearizeAsGain=on  AntiWindupMode=none  Kb=1  TrackingMode=off  Kt=1  PParamMin=[]  PParamMax=[]  IParamMin=[]  IParamMax=[]  DParamMin=[]  DParamMax=[]  NParamMin=[]  NParamMax=[]  KbParamMin=[]  KbParamMax=[]  KtParamMin=[]  KtParamMax=[]  POutMin=[]  POutMax=[]  IOutMin=[]  IOutMax=[]  DOutMin=[]  DOutMax=[]  NOutMin=[]  NOutMax=[]  KbOutMin=[]  KbOutMax=[]  KtOutMin=[]  KtOutMax=[]  IntegratorOutMin=[]  IntegratorOutMax=[]  FilterOutMin=[]  FilterOutMax=[]  SumOutMin=[]  SumOutMax=[]  SumI1OutMin=[]  SumI1OutMax=[]  SumI2OutMin=[]  SumI2OutMax=[]  SumI3OutMin=[]  SumI3OutMax=[]  SumDOutMin=[]  SumDOutMax=[]  SaturationOutMin=[]  SaturationOutMax=[]  IntegratorContinuousStateAttributes=''  IntegratorStateMustResolveToSignalObject=off  IntegratorRTWStateStorageClass=Auto  FilterContinuousStateAttributes=''  FilterStateMustResolveToSignalObject=off  FilterRTWStateStorageClass=Auto  DifferentiatorICPrevScaledInput=0  DifferentiatorOutMin=[]  DifferentiatorOutMax=[]
  Sum1 : Sum  Inputs=+-
  Sum2 : Sum  Inputs=+-
  de : Scope
  q : Selector  InputPortWidth=5  IndexOptions=Index vector (dialog)  Indices=[3]  OutputSizes=1
  theta : Selector  InputPortWidth=5  IndexOptions=Index vector (dialog)  Indices=[4]  OutputSizes=1
  d_elevator : Outport
  wires:
  theta/1 -> Gain7/1
  q/1 -> Gain6/1
  Gain6/1 -> Sum1/2
  Gain7/1 -> Sum2/2
  PID Controller/1 -> Sum1/1
  Sum2/1 -> PID Controller/1
  Ylon/1 -> theta/1, q/1
  Sum1/1 -> de/1, d_elevator/1
  theta_r/1 -> Sum2/1

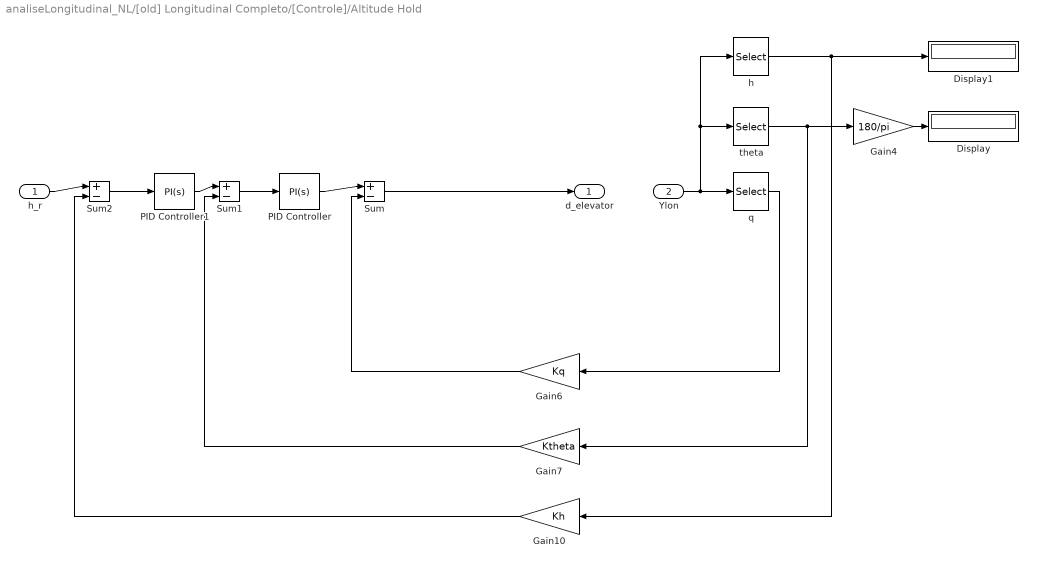
== system analiseLongitudinal_NL/[old] Longitudinal Completo/[Controle]/Altitude Hold ==
  h_r : Inport
  Ylon : Inport  Port=2
  Display : Display
  Display1 : Display
  Gain10 : Gain  Gain=Kh
  Gain4 : Gain  Gain=180/pi
  Gain6 : Gain  Gain=Kq
  Gain7 : Gain  Gain=Ktheta
  PID Controller : simulink/Continuous/PID Controller  Controller=PI  TimeDomain=Continuous-time  SampleTime=-1  IntegratorMethod=Forward Euler  FilterMethod=Forward Euler  Form=Parallel  UseFilter=on  ControllerParametersSource=internal  P=Ctheta.Kp  I=Ctheta.Ki  D=0  N=100  InitialConditionSource=internal  InitialConditionForIntegrator=0  InitialConditionForFilter=0  ExternalReset=none  LimitOutput=off  UpperSaturationLimit=inf  LowerSaturationLimit=-inf  LinearizeAsGain=on  AntiWindupMode=none  Kb=1  TrackingMode=off  Kt=1  PParamMin=[]  PParamMax=[]  IParamMin=[]  IParamMax=[]  DParamMin=[]  DParamMax=[]  NParamMin=[]  NParamMax=[]  KbParamMin=[]  KbParamMax=[]  KtParamMin=[]  KtParamMax=[]  POutMin=[]  POutMax=[]  IOutMin=[]  IOutMax=[]  DOutMin=[]  DOutMax=[]  NOutMin=[]  NOutMax=[]  KbOutMin=[]  KbOutMax=[]  KtOutMin=[]  KtOutMax=[]  IntegratorOutMin=[]  IntegratorOutMax=[]  FilterOutMin=[]  FilterOutMax=[]  SumOutMin=[]  SumOutMax=[]  SumI1OutMin=[]  SumI1OutMax=[]  SumI2OutMin=[]  SumI2OutMax=[]  SumI3OutMin=[]  SumI3OutMax=[]  SumDOutMin=[]  SumDOutMax=[]  SaturationOutMin=[]  SaturationOutMax=[]  IntegratorContinuousStateAttributes=''  IntegratorStateMustResolveToSignalObject=off  IntegratorRTWStateStorageClass=Auto  FilterContinuousStateAttributes=''  FilterStateMustResolveToSignalObject=off  FilterRTWStateStorageClass=Auto  DifferentiatorICPrevScaledInput=0  DifferentiatorOutMin=[]  DifferentiatorOutMax=[]
  PID Controller1 : simulink/Continuous/PID Controller  Controller=PI  TimeDomain=Continuous-time  SampleTime=-1  IntegratorMethod=Forward Euler  FilterMethod=Forward Euler  Form=Parallel  UseFilter=on  ControllerParametersSource=internal  P=Ch.Kp  I=Ch.Ki  D=0  N=100  InitialConditionSource=internal  InitialConditionForIntegrator=0  InitialConditionForFilter=0  ExternalReset=none  LimitOutput=off  UpperSaturationLimit=inf  LowerSaturationLimit=-inf  LinearizeAsGain=on  AntiWindupMode=none  Kb=1  TrackingMode=off  Kt=1  PParamMin=[]  PParamMax=[]  IParamMin=[]  IParamMax=[]  DParamMin=[]  DParamMax=[]  NParamMin=[]  NParamMax=[]  KbParamMin=[]  KbParamMax=[]  KtParamMin=[]  KtParamMax=[]  POutMin=[]  POutMax=[]  IOutMin=[]  IOutMax=[]  DOutMin=[]  DOutMax=[]  NOutMin=[]  NOutMax=[]  KbOutMin=[]  KbOutMax=[]  KtOutMin=[]  KtOutMax=[]  IntegratorOutMin=[]  IntegratorOutMax=[]  FilterOutMin=[]  FilterOutMax=[]  SumOutMin=[]  SumOutMax=[]  SumI1OutMin=[]  SumI1OutMax=[]  SumI2OutMin=[]  SumI2OutMax=[]  SumI3OutMin=[]  SumI3OutMax=[]  SumDOutMin=[]  SumDOutMax=[]  SaturationOutMin=[]  SaturationOutMax=[]  IntegratorContinuousStateAttributes=''  IntegratorStateMustResolveToSignalObject=off  IntegratorRTWStateStorageClass=Auto  FilterContinuousStateAttributes=''  FilterStateMustResolveToSignalObject=off  FilterRTWStateStorageClass=Auto  DifferentiatorICPrevScaledInput=0  DifferentiatorOutMin=[]  DifferentiatorOutMax=[]
  Sum : Sum  Inputs=|+-
  Sum1 : Sum  Inputs=|+-
  Sum2 : Sum  Inputs=|+-
  h : Selector  InputPortWidth=5  IndexOptions=Index vector (dialog)  Indices=[5]  OutputSizes=1
  q : Selector  InputPortWidth=5  IndexOptions=Index vector (dialog)  Indices=[3]  OutputSizes=1
  theta : Selector  InputPortWidth=5  IndexOptions=Index vector (dialog)  Indices=[4]  OutputSizes=1
  d_elevator : Outport
  wires:
  Gain6/1 -> Sum/2
  Gain7/1 -> Sum1/2
  PID Controller/1 -> Sum/1
  Sum1/1 -> PID Controller/1
  PID Controller1/1 -> Sum1/1
  Gain10/1 -> Sum2/2
  Sum2/1 -> PID Controller1/1
  theta/1 -> Gain7/1, Gain4/1
  q/1 -> Gain6/1
  Ylon/1 -> theta/1, h/1, q/1
  h/1 -> Display1/1, Gain10/1
  Sum/1 -> d_elevator/1
  h_r/1 -> Sum2/1
  Gain4/1 -> Display/1

== system analiseLongitudinal_NL/[old] Longitudinal Completo/[Controle]/Controlador Throtle ==
  Vt_r : Inport
  Ylon : Inport  Port=2
  Gain7 : Gain  Gain=KVt
  PID Controller1 : simulink/Continuous/PID Controller  Controller=PI  TimeDomain=Continuous-time  SampleTime=-1  IntegratorMethod=Forward Euler  FilterMethod=Forward Euler  Form=Parallel  UseFilter=on  ControllerParametersSource=internal  P=CVt.Kp  I=CVt.Ki  D=0  N=100  InitialConditionSource=internal  InitialConditionForIntegrator=0  InitialConditionForFilter=0  ExternalReset=none  LimitOutput=off  UpperSaturationLimit=inf  LowerSaturationLimit=-inf  LinearizeAsGain=on  AntiWindupMode=none  Kb=1  TrackingMode=off  Kt=1  PParamMin=[]  PParamMax=[]  IParamMin=[]  IParamMax=[]  DParamMin=[]  DParamMax=[]  NParamMin=[]  NParamMax=[]  KbParamMin=[]  KbParamMax=[]  KtParamMin=[]  KtParamMax=[]  POutMin=[]  POutMax=[]  IOutMin=[]  IOutMax=[]  DOutMin=[]  DOutMax=[]  NOutMin=[]  NOutMax=[]  KbOutMin=[]  KbOutMax=[]  KtOutMin=[]  KtOutMax=[]  IntegratorOutMin=[]  IntegratorOutMax=[]  FilterOutMin=[]  FilterOutMax=[]  SumOutMin=[]  SumOutMax=[]  SumI1OutMin=[]  SumI1OutMax=[]  SumI2OutMin=[]  SumI2OutMax=[]  SumI3OutMin=[]  SumI3OutMax=[]  SumDOutMin=[]  SumDOutMax=[]  SaturationOutMin=[]  SaturationOutMax=[]  IntegratorContinuousStateAttributes=''  IntegratorStateMustResolveToSignalObject=off  IntegratorRTWStateStorageClass=Auto  FilterContinuousStateAttributes=''  FilterStateMustResolveToSignalObject=off  FilterRTWStateStorageClass=Auto  DifferentiatorICPrevScaledInput=0  DifferentiatorOutMin=[]  DifferentiatorOutMax=[]
  Sum : Sum  Inputs=+-
  VT : Selector  InputPortWidth=5  IndexOptions=Index vector (dialog)  Indices=1  OutputSizes=1
  d_throtle : Outport
  wires:
  Sum/1 -> PID Controller1/1
  Vt_r/1 -> Sum/1
  Ylon/1 -> VT/1
  VT/1 -> Gain7/1
  Gain7/1 -> Sum/2
  PID Controller1/1 -> d_throtle/1

== system analiseLongitudinal_NL/[old] Longitudinal Completo/[Controle]/Pitch Attitude Hold ==
  theta_r : Inport
  Ylon : Inport  Port=2
  Display : Display
  Gain6 : Gain  Gain=Kq
  Gain7 : Gain  Gain=Ktheta
  PID Controller : simulink/Continuous/PID Controller  Controller=PI  TimeDomain=Continuous-time  SampleTime=-1  IntegratorMethod=Forward Euler  FilterMethod=Forward Euler  Form=Parallel  UseFilter=on  ControllerParametersSource=internal  P=Ctheta.Kp  I=Ctheta.Ki  D=0  N=100  InitialConditionSource=internal  InitialConditionForIntegrator=0  InitialConditionForFilter=0  ExternalReset=none  LimitOutput=off  UpperSaturationLimit=inf  LowerSaturationLimit=-inf  LinearizeAsGain=on  AntiWindupMode=none  Kb=1  TrackingMode=off  Kt=1  PParamMin=[]  PParamMax=[]  IParamMin=[]  IParamMax=[]  DParamMin=[]  DParamMax=[]  NParamMin=[]  NParamMax=[]  KbParamMin=[]  KbParamMax=[]  KtParamMin=[]  KtParamMax=[]  POutMin=[]  POutMax=[]  IOutMin=[]  IOutMax=[]  DOutMin=[]  DOutMax=[]  NOutMin=[]  NOutMax=[]  KbOutMin=[]  KbOutMax=[]  KtOutMin=[]  KtOutMax=[]  IntegratorOutMin=[]  IntegratorOutMax=[]  FilterOutMin=[]  FilterOutMax=[]  SumOutMin=[]  SumOutMax=[]  SumI1OutMin=[]  SumI1OutMax=[]  SumI2OutMin=[]  SumI2OutMax=[]  SumI3OutMin=[]  SumI3OutMax=[]  SumDOutMin=[]  SumDOutMax=[]  SaturationOutMin=[]  SaturationOutMax=[]  IntegratorContinuousStateAttributes=''  IntegratorStateMustResolveToSignalObject=off  IntegratorRTWStateStorageClass=Auto  FilterContinuousStateAttributes=''  FilterStateMustResolveToSignalObject=off  FilterRTWStateStorageClass=Auto  DifferentiatorICPrevScaledInput=0  DifferentiatorOutMin=[]  DifferentiatorOutMax=[]
  Sum1 : Sum  Inputs=+-
  Sum2 : Sum  Inputs=+-
  de : Scope
  q : Selector  InputPortWidth=5  IndexOptions=Index vector (dialog)  Indices=[3]  OutputSizes=1
  theta : Selector  InputPortWidth=5  IndexOptions=Index vector (dialog)  Indices=[4]  OutputSizes=1
  d_elevator : Outport
  wires:
  theta/1 -> Gain7/1
  q/1 -> Gain6/1
  Gain6/1 -> Sum1/2
  Gain7/1 -> Sum2/2
  PID Controller/1 -> Sum1/1
  Sum2/1 -> PID Controller/1
  Ylon/1 -> Display/1, theta/1, q/1
  Sum1/1 -> de/1, d_elevator/1
  theta_r/1 -> Sum2/1

== system analiseLongitudinal_NL/[old] Longitudinal Completo/[Controle]/else ==
  h_r : Inport
  Yi : Inport  Port=2
  Abs : Abs
  Constant : Constant  Value=0
  Constant1 : Constant  Value=0
  Sum : Sum  Inputs=|+-
  Switch : Switch  Criteria=u2 > Threshold  Threshold=5
  Switch1 : Switch  Criteria=u2 > Threshold  Threshold=5
  VT_r1 : Selector  InputPortWidth=5  IndexOptions=Index vector (dialog)  Indices=[5]  OutputSizes=1
  hr : Outport
  Y : Outport  Port=2
  wires:
  Abs/1 -> Switch1/2, Switch/2
  Yi/1 -> Switch1/3, VT_r1/1
  Switch/1 -> hr/1
  Sum/1 -> Abs/1
  Switch1/1 -> Y/1
  Constant/1 -> Switch/1
  Constant1/1 -> Switch1/1
  h_r/1 -> Sum/1, Switch/3
  VT_r1/1 -> Sum/2

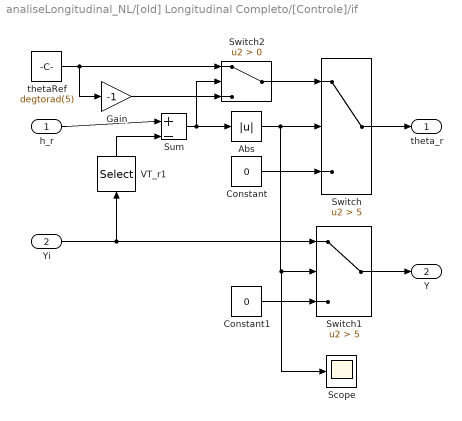
== system analiseLongitudinal_NL/[old] Longitudinal Completo/[Controle]/if ==
  h_r : Inport
  Yi : Inport  Port=2
  Abs : Abs
  Constant : Constant  Value=0
  Constant1 : Constant  Value=0
  Gain : Gain  Gain=-1
  Scope : Scope
  Sum : Sum  Inputs=|+-
  Switch : Switch  Criteria=u2 > Threshold  Threshold=5
  Switch1 : Switch  Criteria=u2 > Threshold  Threshold=5
  Switch2 : Switch  Criteria=u2 > Threshold
  VT_r1 : Selector  InputPortWidth=5  IndexOptions=Index vector (dialog)  Indices=[5]  OutputSizes=1
  thetaRef : Constant  Value=degtorad(5)
  theta_r : Outport
  Y : Outport  Port=2
  wires:
  Abs/1 -> Scope/1, Switch1/2, Switch/2
  Switch/1 -> theta_r/1
  h_r/1 -> Sum/1
  Switch1/1 -> Y/1
  Constant/1 -> Switch/3
  Yi/1 -> VT_r1/1, Switch1/1
  Constant1/1 -> Switch1/3
  Gain/1 -> Switch2/3
  thetaRef/1 -> Gain/1, Switch2/1
  Switch2/1 -> Switch/1
  VT_r1/1 -> Sum/2
  Sum/1 -> Switch2/2, Abs/1
